simulink model "pattern3x3_training_2023noclock"  (R2024a)
settings: Solver=FixedStepAuto  StartTime=0.0  StopTime=2  FixedStep=0.000005  RelTol=1e-3
model workspace (MAT data in the model file):
  part1_v1 = 1
values from neighbouring files (symbols this model uses):
  full_pattern = load('Pattern4_250.CSV')    [model_setup4.m]
  max_weight2 = 255    [model_setup4.m]
  min_weight2 = 150    [model_setup4.m]
  Th_control_time2 = 0.02    [model_setup4.m]    (also in model_setup_test.m = 2)
  Th_minus_count2 = 10    [model_setup4.m]    (also in model_setup_test.m = 5)
  Th_plus_count2 = 20    [model_setup4.m]    (also in model_setup_test.m)
libraries: simulink x1
(part 4 of 9)

== system pattern3x3_training_2023noclock/Synapse35 ==
  note: weight 초기값
  note: pre spike trace
  note: weight 최댓값
  note: STDP
  note: Synapse
  note: weight 최솟값
  note: post spike trace
  note: 기존 weight + STDP 변화량
  note: weight RC 감소
  Pre_spike : Inport
  addr : Inport  Port=2
  Post_spike : Inport  Port=3
  Add1 : Sum
  Clock1 : Subsystem
  Clock2 : Subsystem
  Clock3 : Subsystem
  Delay1 : Delay  DelayLength=1  SampleTime=0.00001
  Exp : Math
  Exp1 : Math
  From Workspace : FromWorkspace  VariableName=Rand_var
  From Workspace1 : FromWorkspace  VariableName=min_weight
  From Workspace2 : FromWorkspace  VariableName=max_weight
  From Workspace3 : FromWorkspace  VariableName=synapse_weight_rc_s
  From Workspace4 : FromWorkspace  VariableName=synapse_weight_rc_l
  From Workspace6 : FromWorkspace  VariableName=initial_LTP
  From Workspace7 : FromWorkspace  VariableName=initial_LTD
  From Workspace8 : FromWorkspace  VariableName=RC_LTP
  From Workspace9 : FromWorkspace  VariableName=RC_LTD
  Gain1 : Gain  Gain=-1
  MATLAB Function1 : MATLAB Function  TreatAsAtomicUnit=on
  Memory1 : Memory
  Memory2 : Memory
  OR : Logic  Operator=OR  IconShape=distinctive  AllPortsSameDT=off  OutDataTypeStr=boolean
  Product{,1..6} (7 alike) : Product
  Scope1 : Scope  NumInputPorts=4
  Scope2 : Scope  NumInputPorts=5
  Scope3 : Scope  NumInputPorts=2
  Scope5 : Scope  NumInputPorts=3
  Scope6 : Scope  NumInputPorts=3
  Scope7 : Scope  NumInputPorts=3
  Scope8 : Scope  NumInputPorts=4
  Subsystem : Subsystem
  Switch : Switch  Threshold=max_weight2  SaturateOnIntegerOverflow=off  InputSameDT=off
  Switch1 : Switch  Criteria=u2 > Threshold  Threshold=min_weight2  SaturateOnIntegerOverflow=off  InputSameDT=off
  rc_add1 : MATLAB Function  TreatAsAtomicUnit=on
  rc_add2 : MATLAB Function  TreatAsAtomicUnit=on
  Weight : Outport
  Spike_out : Outport  Port=2
  Weight_out : Outport  Port=3
  wires:
  Switch1/1 -> Scope7/3, Product/2, Weight_out/1, Scope5/3, Scope3/1, Delay1/1
  Product/1 -> Memory1/1
  addr/1 -> MATLAB Function1/2(synapse_num)
  Post_spike/1 -> Scope2/4, Memory2/1
  Clock1/1(T) -> rc_add2/1(tx)
  Clock2/1(T) -> Scope2/3, rc_add1/1(ty)
  Delay1/1 -> Scope3/2, Subsystem/2(before_weight), Scope6/3
  Memory1/1 -> Weight/1, Scope5/2
  From Workspace7/1 -> rc_add1/2(initial_LTD)
  From Workspace9/1 -> rc_add1/3(RC_LTD)
  From Workspace6/1 -> rc_add2/2(initial_LTP)
  From Workspace8/1 -> rc_add2/3(RC_LTP)
  Product6/1 -> Scope1/4, Add1/2
  Product5/1 -> Scope1/3, Add1/1
  Add1/1 -> Subsystem/1(delta_weight), Scope2/1, Scope6/1
  From Workspace2/1 -> Product3/2
  Product2/1 -> Exp1/1
  Gain1/1 -> Product1/2, Product2/1
  From Workspace1/1 -> Switch1/3
  Exp1/1 -> Scope8/2, Product4/2
  Switch/1 -> Scope8/4, Switch1/2, Scope7/2, Switch1/1
  From Workspace3/1 -> Product2/2
  Product3/1 -> Switch/1
  Exp/1 -> Product3/1
  Clock3/1(T) -> Gain1/1
  Product1/1 -> Exp/1
  MATLAB Function1/1(y) -> Scope6/2, Product4/1, Scope7/1, Switch/2, Scope8/1
  From Workspace4/1 -> Product1/1
  From Workspace/1 -> MATLAB Function1/1(init_weight)
  Product4/1 -> Scope8/3, Switch/3
  Subsystem/1(weight) -> MATLAB Function1/3(before_weight)
  rc_add2/1(pre_trace) -> Product5/1
  rc_add1/1(post_trace) -> Product6/2
  OR/1 -> Subsystem/Trigger
  Memory2/1 -> OR/2, Scope1/2, Product5/2, Clock2/1("Reset "), Scope2/5
  Pre_spike/1 -> OR/1, Scope1/1, Scope5/1, Spike_out/1, Product/1, Clock3/1("Reset "), Clock1/1("Reset "), Product6/1, Scope2/2

== system pattern3x3_training_2023noclock/Synapse36 ==
  note: weight 초기값
  note: pre spike trace
  note: weight 최댓값
  note: STDP
  note: Synapse
  note: weight 최솟값
  note: post spike trace
  note: 기존 weight + STDP 변화량
  note: weight RC 감소
  Pre_spike : Inport
  addr : Inport  Port=2
  Post_spike : Inport  Port=3
  Add1 : Sum
  Clock1 : Subsystem
  Clock2 : Subsystem
  Clock3 : Subsystem
  Delay1 : Delay  DelayLength=1  SampleTime=0.00001
  Exp : Math
  Exp1 : Math
  From Workspace : FromWorkspace  VariableName=Rand_var
  From Workspace1 : FromWorkspace  VariableName=min_weight
  From Workspace2 : FromWorkspace  VariableName=max_weight
  From Workspace3 : FromWorkspace  VariableName=synapse_weight_rc_s
  From Workspace4 : FromWorkspace  VariableName=synapse_weight_rc_l
  From Workspace6 : FromWorkspace  VariableName=initial_LTP
  From Workspace7 : FromWorkspace  VariableName=initial_LTD
  From Workspace8 : FromWorkspace  VariableName=RC_LTP
  From Workspace9 : FromWorkspace  VariableName=RC_LTD
  Gain1 : Gain  Gain=-1
  MATLAB Function1 : MATLAB Function  TreatAsAtomicUnit=on
  Memory1 : Memory
  Memory2 : Memory
  OR : Logic  Operator=OR  IconShape=distinctive  AllPortsSameDT=off  OutDataTypeStr=boolean
  Product{,1..6} (7 alike) : Product
  Scope1 : Scope  NumInputPorts=4
  Scope2 : Scope  NumInputPorts=5
  Scope3 : Scope  NumInputPorts=2
  Scope5 : Scope  NumInputPorts=3
  Scope6 : Scope  NumInputPorts=3
  Scope7 : Scope  NumInputPorts=3
  Scope8 : Scope  NumInputPorts=4
  Subsystem : Subsystem
  Switch : Switch  Threshold=max_weight2  SaturateOnIntegerOverflow=off  InputSameDT=off
  Switch1 : Switch  Criteria=u2 > Threshold  Threshold=min_weight2  SaturateOnIntegerOverflow=off  InputSameDT=off
  rc_add1 : MATLAB Function  TreatAsAtomicUnit=on
  rc_add2 : MATLAB Function  TreatAsAtomicUnit=on
  Weight : Outport
  Spike_out : Outport  Port=2
  Weight_out : Outport  Port=3
  wires:
  Switch1/1 -> Scope7/3, Product/2, Weight_out/1, Scope5/3, Scope3/1, Delay1/1
  Product/1 -> Memory1/1
  addr/1 -> MATLAB Function1/2(synapse_num)
  Post_spike/1 -> Scope2/4, Memory2/1
  Clock1/1(T) -> rc_add2/1(tx)
  Clock2/1(T) -> Scope2/3, rc_add1/1(ty)
  Delay1/1 -> Scope3/2, Subsystem/2(before_weight), Scope6/3
  Memory1/1 -> Weight/1, Scope5/2
  From Workspace7/1 -> rc_add1/2(initial_LTD)
  From Workspace9/1 -> rc_add1/3(RC_LTD)
  From Workspace6/1 -> rc_add2/2(initial_LTP)
  From Workspace8/1 -> rc_add2/3(RC_LTP)
  Product6/1 -> Scope1/4, Add1/2
  Product5/1 -> Scope1/3, Add1/1
  Add1/1 -> Subsystem/1(delta_weight), Scope2/1, Scope6/1
  From Workspace2/1 -> Product3/2
  Product2/1 -> Exp1/1
  Gain1/1 -> Product1/2, Product2/1
  From Workspace1/1 -> Switch1/3
  Exp1/1 -> Scope8/2, Product4/2
  Switch/1 -> Scope8/4, Switch1/2, Scope7/2, Switch1/1
  From Workspace3/1 -> Product2/2
  Product3/1 -> Switch/1
  Exp/1 -> Product3/1
  Clock3/1(T) -> Gain1/1
  Product1/1 -> Exp/1
  MATLAB Function1/1(y) -> Scope6/2, Product4/1, Scope7/1, Switch/2, Scope8/1
  From Workspace4/1 -> Product1/1
  From Workspace/1 -> MATLAB Function1/1(init_weight)
  Product4/1 -> Scope8/3, Switch/3
  Subsystem/1(weight) -> MATLAB Function1/3(before_weight)
  rc_add2/1(pre_trace) -> Product5/1
  rc_add1/1(post_trace) -> Product6/2
  OR/1 -> Subsystem/Trigger
  Memory2/1 -> OR/2, Scope1/2, Product5/2, Clock2/1("Reset "), Scope2/5
  Pre_spike/1 -> OR/1, Scope1/1, Scope5/1, Spike_out/1, Product/1, Clock3/1("Reset "), Clock1/1("Reset "), Product6/1, Scope2/2

== system pattern3x3_training_2023noclock/Synapse4 ==
  note: weight 초기값
  note: pre spike trace
  note: weight 최댓값
  note: STDP
  note: Synapse
  note: weight 최솟값
  note: post spike trace
  note: 기존 weight + STDP 변화량
  note: weight RC 감소
  Pre_spike : Inport
  addr : Inport  Port=2
  Post_spike : Inport  Port=3
  Add1 : Sum
  Clock1 : Subsystem
  Clock2 : Subsystem
  Clock3 : Subsystem
  Delay1 : Delay  DelayLength=1  SampleTime=0.00001
  Exp : Math
  Exp1 : Math
  From Workspace : FromWorkspace  VariableName=Rand_var
  From Workspace1 : FromWorkspace  VariableName=min_weight
  From Workspace2 : FromWorkspace  VariableName=max_weight
  From Workspace3 : FromWorkspace  VariableName=synapse_weight_rc_s
  From Workspace4 : FromWorkspace  VariableName=synapse_weight_rc_l
  From Workspace6 : FromWorkspace  VariableName=initial_LTP
  From Workspace7 : FromWorkspace  VariableName=initial_LTD
  From Workspace8 : FromWorkspace  VariableName=RC_LTP
  From Workspace9 : FromWorkspace  VariableName=RC_LTD
  Gain1 : Gain  Gain=-1
  MATLAB Function1 : MATLAB Function  TreatAsAtomicUnit=on
  Memory1 : Memory
  Memory2 : Memory
  OR : Logic  Operator=OR  IconShape=distinctive  AllPortsSameDT=off  OutDataTypeStr=boolean
  Product{,1..6} (7 alike) : Product
  Scope1 : Scope  NumInputPorts=4
  Scope2 : Scope  NumInputPorts=5
  Scope3 : Scope  NumInputPorts=2
  Scope5 : Scope  NumInputPorts=3
  Scope6 : Scope  NumInputPorts=3
  Scope7 : Scope  NumInputPorts=3
  Scope8 : Scope  NumInputPorts=4
  Subsystem : Subsystem
  Switch : Switch  Threshold=max_weight2  SaturateOnIntegerOverflow=off  InputSameDT=off
  Switch1 : Switch  Criteria=u2 > Threshold  Threshold=min_weight2  SaturateOnIntegerOverflow=off  InputSameDT=off
  rc_add1 : MATLAB Function  TreatAsAtomicUnit=on
  rc_add2 : MATLAB Function  TreatAsAtomicUnit=on
  Weight : Outport
  Spike_out : Outport  Port=2
  Weight_out : Outport  Port=3
  wires:
  Switch1/1 -> Scope7/3, Product/2, Weight_out/1, Scope5/3, Scope3/1, Delay1/1
  Product/1 -> Memory1/1
  addr/1 -> MATLAB Function1/2(synapse_num)
  Post_spike/1 -> Scope2/4, Memory2/1
  Clock1/1(T) -> rc_add2/1(tx)
  Clock2/1(T) -> Scope2/3, rc_add1/1(ty)
  Delay1/1 -> Scope3/2, Subsystem/2(before_weight), Scope6/3
  Memory1/1 -> Weight/1, Scope5/2
  From Workspace7/1 -> rc_add1/2(initial_LTD)
  From Workspace9/1 -> rc_add1/3(RC_LTD)
  From Workspace6/1 -> rc_add2/2(initial_LTP)
  From Workspace8/1 -> rc_add2/3(RC_LTP)
  Product6/1 -> Scope1/4, Add1/2
  Product5/1 -> Scope1/3, Add1/1
  Add1/1 -> Subsystem/1(delta_weight), Scope2/1, Scope6/1
  From Workspace2/1 -> Product3/2
  Product2/1 -> Exp1/1
  Gain1/1 -> Product1/2, Product2/1
  From Workspace1/1 -> Switch1/3
  Exp1/1 -> Scope8/2, Product4/2
  Switch/1 -> Scope8/4, Switch1/2, Scope7/2, Switch1/1
  From Workspace3/1 -> Product2/2
  Product3/1 -> Switch/1
  Exp/1 -> Product3/1
  Clock3/1(T) -> Gain1/1
  Product1/1 -> Exp/1
  MATLAB Function1/1(y) -> Scope6/2, Product4/1, Scope7/1, Switch/2, Scope8/1
  From Workspace4/1 -> Product1/1
  From Workspace/1 -> MATLAB Function1/1(init_weight)
  Product4/1 -> Scope8/3, Switch/3
  Subsystem/1(weight) -> MATLAB Function1/3(before_weight)
  rc_add2/1(pre_trace) -> Product5/1
  rc_add1/1(post_trace) -> Product6/2
  OR/1 -> Subsystem/Trigger
  Memory2/1 -> OR/2, Scope1/2, Product5/2, Clock2/1("Reset "), Scope2/5
  Pre_spike/1 -> OR/1, Scope1/1, Scope5/1, Spike_out/1, Product/1, Clock3/1("Reset "), Clock1/1("Reset "), Product6/1, Scope2/2

== system pattern3x3_training_2023noclock/Synapse5 ==
  note: weight 초기값
  note: pre spike trace
  note: weight 최댓값
  note: STDP
  note: Synapse
  note: weight 최솟값
  note: post spike trace
  note: 기존 weight + STDP 변화량
  note: weight RC 감소
  Pre_spike : Inport
  addr : Inport  Port=2
  Post_spike : Inport  Port=3
  Add1 : Sum
  Clock1 : Subsystem
  Clock2 : Subsystem
  Clock3 : Subsystem
  Delay1 : Delay  DelayLength=1  SampleTime=0.00001
  Exp : Math
  Exp1 : Math
  From Workspace : FromWorkspace  VariableName=Rand_var
  From Workspace1 : FromWorkspace  VariableName=min_weight
  From Workspace2 : FromWorkspace  VariableName=max_weight
  From Workspace3 : FromWorkspace  VariableName=synapse_weight_rc_s
  From Workspace4 : FromWorkspace  VariableName=synapse_weight_rc_l
  From Workspace6 : FromWorkspace  VariableName=initial_LTP
  From Workspace7 : FromWorkspace  VariableName=initial_LTD
  From Workspace8 : FromWorkspace  VariableName=RC_LTP
  From Workspace9 : FromWorkspace  VariableName=RC_LTD
  Gain1 : Gain  Gain=-1
  MATLAB Function1 : MATLAB Function  TreatAsAtomicUnit=on
  Memory1 : Memory
  Memory2 : Memory
  OR : Logic  Operator=OR  IconShape=distinctive  AllPortsSameDT=off  OutDataTypeStr=boolean
  Product{,1..6} (7 alike) : Product
  Scope1 : Scope  NumInputPorts=4
  Scope2 : Scope  NumInputPorts=5
  Scope3 : Scope  NumInputPorts=2
  Scope5 : Scope  NumInputPorts=3
  Scope6 : Scope  NumInputPorts=3
  Scope7 : Scope  NumInputPorts=3
  Scope8 : Scope  NumInputPorts=4
  Subsystem : Subsystem
  Switch : Switch  Threshold=max_weight2  SaturateOnIntegerOverflow=off  InputSameDT=off
  Switch1 : Switch  Criteria=u2 > Threshold  Threshold=min_weight2  SaturateOnIntegerOverflow=off  InputSameDT=off
  rc_add1 : MATLAB Function  TreatAsAtomicUnit=on
  rc_add2 : MATLAB Function  TreatAsAtomicUnit=on
  Weight : Outport
  Spike_out : Outport  Port=2
  Weight_out : Outport  Port=3
  wires:
  Switch1/1 -> Scope7/3, Product/2, Weight_out/1, Scope5/3, Scope3/1, Delay1/1
  Product/1 -> Memory1/1
  addr/1 -> MATLAB Function1/2(synapse_num)
  Post_spike/1 -> Scope2/4, Memory2/1
  Clock1/1(T) -> rc_add2/1(tx)
  Clock2/1(T) -> Scope2/3, rc_add1/1(ty)
  Delay1/1 -> Scope3/2, Subsystem/2(before_weight), Scope6/3
  Memory1/1 -> Weight/1, Scope5/2
  From Workspace7/1 -> rc_add1/2(initial_LTD)
  From Workspace9/1 -> rc_add1/3(RC_LTD)
  From Workspace6/1 -> rc_add2/2(initial_LTP)
  From Workspace8/1 -> rc_add2/3(RC_LTP)
  Product6/1 -> Scope1/4, Add1/2
  Product5/1 -> Scope1/3, Add1/1
  Add1/1 -> Subsystem/1(delta_weight), Scope2/1, Scope6/1
  From Workspace2/1 -> Product3/2
  Product2/1 -> Exp1/1
  Gain1/1 -> Product1/2, Product2/1
  From Workspace1/1 -> Switch1/3
  Exp1/1 -> Scope8/2, Product4/2
  Switch/1 -> Scope8/4, Switch1/2, Scope7/2, Switch1/1
  From Workspace3/1 -> Product2/2
  Product3/1 -> Switch/1
  Exp/1 -> Product3/1
  Clock3/1(T) -> Gain1/1
  Product1/1 -> Exp/1
  MATLAB Function1/1(y) -> Scope6/2, Product4/1, Scope7/1, Switch/2, Scope8/1
  From Workspace4/1 -> Product1/1
  From Workspace/1 -> MATLAB Function1/1(init_weight)
  Product4/1 -> Scope8/3, Switch/3
  Subsystem/1(weight) -> MATLAB Function1/3(before_weight)
  rc_add2/1(pre_trace) -> Product5/1
  rc_add1/1(post_trace) -> Product6/2
  OR/1 -> Subsystem/Trigger
  Memory2/1 -> OR/2, Scope1/2, Product5/2, Clock2/1("Reset "), Scope2/5
  Pre_spike/1 -> OR/1, Scope1/1, Scope5/1, Spike_out/1, Product/1, Clock3/1("Reset "), Clock1/1("Reset "), Product6/1, Scope2/2

== system pattern3x3_training_2023noclock/Synapse6 ==
  note: weight 초기값
  note: pre spike trace
  note: weight 최댓값
  note: STDP
  note: Synapse
  note: weight 최솟값
  note: post spike trace
  note: 기존 weight + STDP 변화량
  note: weight RC 감소
  Pre_spike : Inport
  addr : Inport  Port=2
  Post_spike : Inport  Port=3
  Add1 : Sum
  Clock1 : Subsystem
  Clock2 : Subsystem
  Clock3 : Subsystem
  Delay1 : Delay  DelayLength=1  SampleTime=0.00001
  Exp : Math
  Exp1 : Math
  From Workspace : FromWorkspace  VariableName=Rand_var
  From Workspace1 : FromWorkspace  VariableName=min_weight
  From Workspace2 : FromWorkspace  VariableName=max_weight
  From Workspace3 : FromWorkspace  VariableName=synapse_weight_rc_s
  From Workspace4 : FromWorkspace  VariableName=synapse_weight_rc_l
  From Workspace6 : FromWorkspace  VariableName=initial_LTP
  From Workspace7 : FromWorkspace  VariableName=initial_LTD
  From Workspace8 : FromWorkspace  VariableName=RC_LTP
  From Workspace9 : FromWorkspace  VariableName=RC_LTD
  Gain1 : Gain  Gain=-1
  MATLAB Function1 : MATLAB Function  TreatAsAtomicUnit=on
  Memory1 : Memory
  Memory2 : Memory
  OR : Logic  Operator=OR  IconShape=distinctive  AllPortsSameDT=off  OutDataTypeStr=boolean
  Product{,1..6} (7 alike) : Product
  Scope1 : Scope  NumInputPorts=4
  Scope2 : Scope  NumInputPorts=5
  Scope3 : Scope  NumInputPorts=2
  Scope5 : Scope  NumInputPorts=3
  Scope6 : Scope  NumInputPorts=3
  Scope7 : Scope  NumInputPorts=3
  Scope8 : Scope  NumInputPorts=4
  Subsystem : Subsystem
  Switch : Switch  Threshold=max_weight2  SaturateOnIntegerOverflow=off  InputSameDT=off
  Switch1 : Switch  Criteria=u2 > Threshold  Threshold=min_weight2  SaturateOnIntegerOverflow=off  InputSameDT=off
  rc_add1 : MATLAB Function  TreatAsAtomicUnit=on
  rc_add2 : MATLAB Function  TreatAsAtomicUnit=on
  Weight : Outport
  Spike_out : Outport  Port=2
  Weight_out : Outport  Port=3
  wires:
  Switch1/1 -> Scope7/3, Product/2, Weight_out/1, Scope5/3, Scope3/1, Delay1/1
  Product/1 -> Memory1/1
  addr/1 -> MATLAB Function1/2(synapse_num)
  Post_spike/1 -> Scope2/4, Memory2/1
  Clock1/1(T) -> rc_add2/1(tx)
  Clock2/1(T) -> Scope2/3, rc_add1/1(ty)
  Delay1/1 -> Scope3/2, Subsystem/2(before_weight), Scope6/3
  Memory1/1 -> Weight/1, Scope5/2
  From Workspace7/1 -> rc_add1/2(initial_LTD)
  From Workspace9/1 -> rc_add1/3(RC_LTD)
  From Workspace6/1 -> rc_add2/2(initial_LTP)
  From Workspace8/1 -> rc_add2/3(RC_LTP)
  Product6/1 -> Scope1/4, Add1/2
  Product5/1 -> Scope1/3, Add1/1
  Add1/1 -> Subsystem/1(delta_weight), Scope2/1, Scope6/1
  From Workspace2/1 -> Product3/2
  Product2/1 -> Exp1/1
  Gain1/1 -> Product1/2, Product2/1
  From Workspace1/1 -> Switch1/3
  Exp1/1 -> Scope8/2, Product4/2
  Switch/1 -> Scope8/4, Switch1/2, Scope7/2, Switch1/1
  From Workspace3/1 -> Product2/2
  Product3/1 -> Switch/1
  Exp/1 -> Product3/1
  Clock3/1(T) -> Gain1/1
  Product1/1 -> Exp/1
  MATLAB Function1/1(y) -> Scope6/2, Product4/1, Scope7/1, Switch/2, Scope8/1
  From Workspace4/1 -> Product1/1
  From Workspace/1 -> MATLAB Function1/1(init_weight)
  Product4/1 -> Scope8/3, Switch/3
  Subsystem/1(weight) -> MATLAB Function1/3(before_weight)
  rc_add2/1(pre_trace) -> Product5/1
  rc_add1/1(post_trace) -> Product6/2
  OR/1 -> Subsystem/Trigger
  Memory2/1 -> OR/2, Scope1/2, Product5/2, Clock2/1("Reset "), Scope2/5
  Pre_spike/1 -> OR/1, Scope1/1, Scope5/1, Spike_out/1, Product/1, Clock3/1("Reset "), Clock1/1("Reset "), Product6/1, Scope2/2

== system pattern3x3_training_2023noclock/Synapse7 ==
  note: weight 초기값
  note: pre spike trace
  note: weight 최댓값
  note: STDP
  note: Synapse
  note: weight 최솟값
  note: post spike trace
  note: 기존 weight + STDP 변화량
  note: weight RC 감소
  Pre_spike : Inport
  addr : Inport  Port=2
  Post_spike : Inport  Port=3
  Add1 : Sum
  Clock1 : Subsystem
  Clock2 : Subsystem
  Clock3 : Subsystem
  Delay1 : Delay  DelayLength=1  SampleTime=0.00001
  Exp : Math
  Exp1 : Math
  From Workspace : FromWorkspace  VariableName=Rand_var
  From Workspace1 : FromWorkspace  VariableName=min_weight
  From Workspace2 : FromWorkspace  VariableName=max_weight
  From Workspace3 : FromWorkspace  VariableName=synapse_weight_rc_s
  From Workspace4 : FromWorkspace  VariableName=synapse_weight_rc_l
  From Workspace6 : FromWorkspace  VariableName=initial_LTP
  From Workspace7 : FromWorkspace  VariableName=initial_LTD
  From Workspace8 : FromWorkspace  VariableName=RC_LTP
  From Workspace9 : FromWorkspace  VariableName=RC_LTD
  Gain1 : Gain  Gain=-1
  MATLAB Function1 : MATLAB Function  TreatAsAtomicUnit=on
  Memory1 : Memory
  Memory2 : Memory
  OR : Logic  Operator=OR  IconShape=distinctive  AllPortsSameDT=off  OutDataTypeStr=boolean
  Product{,1..6} (7 alike) : Product
  Scope1 : Scope  NumInputPorts=4
  Scope2 : Scope  NumInputPorts=5
  Scope3 : Scope  NumInputPorts=2
  Scope5 : Scope  NumInputPorts=3
  Scope6 : Scope  NumInputPorts=3
  Scope7 : Scope  NumInputPorts=3
  Scope8 : Scope  NumInputPorts=4
  Subsystem : Subsystem
  Switch : Switch  Threshold=max_weight2  SaturateOnIntegerOverflow=off  InputSameDT=off
  Switch1 : Switch  Criteria=u2 > Threshold  Threshold=min_weight2  SaturateOnIntegerOverflow=off  InputSameDT=off
  rc_add1 : MATLAB Function  TreatAsAtomicUnit=on
  rc_add2 : MATLAB Function  TreatAsAtomicUnit=on
  Weight : Outport
  Spike_out : Outport  Port=2
  Weight_out : Outport  Port=3
  wires:
  Switch1/1 -> Scope7/3, Product/2, Weight_out/1, Scope5/3, Scope3/1, Delay1/1
  Product/1 -> Memory1/1
  addr/1 -> MATLAB Function1/2(synapse_num)
  Post_spike/1 -> Scope2/4, Memory2/1
  Clock1/1(T) -> rc_add2/1(tx)
  Clock2/1(T) -> Scope2/3, rc_add1/1(ty)
  Delay1/1 -> Scope3/2, Subsystem/2(before_weight), Scope6/3
  Memory1/1 -> Weight/1, Scope5/2
  From Workspace7/1 -> rc_add1/2(initial_LTD)
  From Workspace9/1 -> rc_add1/3(RC_LTD)
  From Workspace6/1 -> rc_add2/2(initial_LTP)
  From Workspace8/1 -> rc_add2/3(RC_LTP)
  Product6/1 -> Scope1/4, Add1/2
  Product5/1 -> Scope1/3, Add1/1
  Add1/1 -> Subsystem/1(delta_weight), Scope2/1, Scope6/1
  From Workspace2/1 -> Product3/2
  Product2/1 -> Exp1/1
  Gain1/1 -> Product1/2, Product2/1
  From Workspace1/1 -> Switch1/3
  Exp1/1 -> Scope8/2, Product4/2
  Switch/1 -> Scope8/4, Switch1/2, Scope7/2, Switch1/1
  From Workspace3/1 -> Product2/2
  Product3/1 -> Switch/1
  Exp/1 -> Product3/1
  Clock3/1(T) -> Gain1/1
  Product1/1 -> Exp/1
  MATLAB Function1/1(y) -> Scope6/2, Product4/1, Scope7/1, Switch/2, Scope8/1
  From Workspace4/1 -> Product1/1
  From Workspace/1 -> MATLAB Function1/1(init_weight)
  Product4/1 -> Scope8/3, Switch/3
  Subsystem/1(weight) -> MATLAB Function1/3(before_weight)
  rc_add2/1(pre_trace) -> Product5/1
  rc_add1/1(post_trace) -> Product6/2
  OR/1 -> Subsystem/Trigger
  Memory2/1 -> OR/2, Scope1/2, Product5/2, Clock2/1("Reset "), Scope2/5
  Pre_spike/1 -> OR/1, Scope1/1, Scope5/1, Spike_out/1, Product/1, Clock3/1("Reset "), Clock1/1("Reset "), Product6/1, Scope2/2

== system pattern3x3_training_2023noclock/Synapse8 ==
  note: weight 초기값
  note: pre spike trace
  note: weight 최댓값
  note: STDP
  note: Synapse
  note: weight 최솟값
  note: post spike trace
  note: 기존 weight + STDP 변화량
  note: weight RC 감소
  Pre_spike : Inport
  addr : Inport  Port=2
  Post_spike : Inport  Port=3
  Add1 : Sum
  Clock1 : Subsystem
  Clock2 : Subsystem
  Clock3 : Subsystem
  Delay1 : Delay  DelayLength=1  SampleTime=0.00001
  Exp : Math
  Exp1 : Math
  From Workspace : FromWorkspace  VariableName=Rand_var
  From Workspace1 : FromWorkspace  VariableName=min_weight
  From Workspace2 : FromWorkspace  VariableName=max_weight
  From Workspace3 : FromWorkspace  VariableName=synapse_weight_rc_s
  From Workspace4 : FromWorkspace  VariableName=synapse_weight_rc_l
  From Workspace6 : FromWorkspace  VariableName=initial_LTP
  From Workspace7 : FromWorkspace  VariableName=initial_LTD
  From Workspace8 : FromWorkspace  VariableName=RC_LTP
  From Workspace9 : FromWorkspace  VariableName=RC_LTD
  Gain1 : Gain  Gain=-1
  MATLAB Function1 : MATLAB Function  TreatAsAtomicUnit=on
  Memory1 : Memory
  Memory2 : Memory
  OR : Logic  Operator=OR  IconShape=distinctive  AllPortsSameDT=off  OutDataTypeStr=boolean
  Product{,1..6} (7 alike) : Product
  Scope1 : Scope  NumInputPorts=4
  Scope2 : Scope  NumInputPorts=5
  Scope3 : Scope  NumInputPorts=2
  Scope5 : Scope  NumInputPorts=3
  Scope6 : Scope  NumInputPorts=3
  Scope7 : Scope  NumInputPorts=3
  Scope8 : Scope  NumInputPorts=4
  Subsystem : Subsystem
  Switch : Switch  Threshold=max_weight2  SaturateOnIntegerOverflow=off  InputSameDT=off
  Switch1 : Switch  Criteria=u2 > Threshold  Threshold=min_weight2  SaturateOnIntegerOverflow=off  InputSameDT=off
  rc_add1 : MATLAB Function  TreatAsAtomicUnit=on
  rc_add2 : MATLAB Function  TreatAsAtomicUnit=on
  Weight : Outport
  Spike_out : Outport  Port=2
  Weight_out : Outport  Port=3
  wires:
  Switch1/1 -> Scope7/3, Product/2, Weight_out/1, Scope5/3, Scope3/1, Delay1/1
  Product/1 -> Memory1/1
  addr/1 -> MATLAB Function1/2(synapse_num)
  Post_spike/1 -> Scope2/4, Memory2/1
  Clock1/1(T) -> rc_add2/1(tx)
  Clock2/1(T) -> Scope2/3, rc_add1/1(ty)
  Delay1/1 -> Scope3/2, Subsystem/2(before_weight), Scope6/3
  Memory1/1 -> Weight/1, Scope5/2
  From Workspace7/1 -> rc_add1/2(initial_LTD)
  From Workspace9/1 -> rc_add1/3(RC_LTD)
  From Workspace6/1 -> rc_add2/2(initial_LTP)
  From Workspace8/1 -> rc_add2/3(RC_LTP)
  Product6/1 -> Scope1/4, Add1/2
  Product5/1 -> Scope1/3, Add1/1
  Add1/1 -> Subsystem/1(delta_weight), Scope2/1, Scope6/1
  From Workspace2/1 -> Product3/2
  Product2/1 -> Exp1/1
  Gain1/1 -> Product1/2, Product2/1
  From Workspace1/1 -> Switch1/3
  Exp1/1 -> Scope8/2, Product4/2
  Switch/1 -> Scope8/4, Switch1/2, Scope7/2, Switch1/1
  From Workspace3/1 -> Product2/2
  Product3/1 -> Switch/1
  Exp/1 -> Product3/1
  Clock3/1(T) -> Gain1/1
  Product1/1 -> Exp/1
  MATLAB Function1/1(y) -> Scope6/2, Product4/1, Scope7/1, Switch/2, Scope8/1
  From Workspace4/1 -> Product1/1
  From Workspace/1 -> MATLAB Function1/1(init_weight)
  Product4/1 -> Scope8/3, Switch/3
  Subsystem/1(weight) -> MATLAB Function1/3(before_weight)
  rc_add2/1(pre_trace) -> Product5/1
  rc_add1/1(post_trace) -> Product6/2
  OR/1 -> Subsystem/Trigger
  Memory2/1 -> OR/2, Scope1/2, Product5/2, Clock2/1("Reset "), Scope2/5
  Pre_spike/1 -> OR/1, Scope1/1, Scope5/1, Spike_out/1, Product/1, Clock3/1("Reset "), Clock1/1("Reset "), Product6/1, Scope2/2

== system pattern3x3_training_2023noclock/Synapse9 ==
  note: weight 초기값
  note: pre spike trace
  note: weight 최댓값
  note: STDP
  note: Synapse
  note: weight 최솟값
  note: post spike trace
  note: 기존 weight + STDP 변화량
  note: weight RC 감소
  Pre_spike : Inport
  addr : Inport  Port=2
  Post_spike : Inport  Port=3
  Add1 : Sum
  Clock1 : Subsystem
  Clock2 : Subsystem
  Clock3 : Subsystem
  Delay1 : Delay  DelayLength=1  SampleTime=0.00001
  Exp : Math
  Exp1 : Math
  From Workspace : FromWorkspace  VariableName=Rand_var
  From Workspace1 : FromWorkspace  VariableName=min_weight
  From Workspace2 : FromWorkspace  VariableName=max_weight
  From Workspace3 : FromWorkspace  VariableName=synapse_weight_rc_s
  From Workspace4 : FromWorkspace  VariableName=synapse_weight_rc_l
  From Workspace6 : FromWorkspace  VariableName=initial_LTP
  From Workspace7 : FromWorkspace  VariableName=initial_LTD
  From Workspace8 : FromWorkspace  VariableName=RC_LTP
  From Workspace9 : FromWorkspace  VariableName=RC_LTD
  Gain1 : Gain  Gain=-1
  MATLAB Function1 : MATLAB Function  TreatAsAtomicUnit=on
  Memory1 : Memory
  Memory2 : Memory
  OR : Logic  Operator=OR  IconShape=distinctive  AllPortsSameDT=off  OutDataTypeStr=boolean
  Product{,1..6} (7 alike) : Product
  Scope1 : Scope  NumInputPorts=4
  Scope2 : Scope  NumInputPorts=5
  Scope3 : Scope  NumInputPorts=2
  Scope5 : Scope  NumInputPorts=3
  Scope6 : Scope  NumInputPorts=3
  Scope7 : Scope  NumInputPorts=3
  Scope8 : Scope  NumInputPorts=4
  Subsystem : Subsystem
  Switch : Switch  Threshold=max_weight2  SaturateOnIntegerOverflow=off  InputSameDT=off
  Switch1 : Switch  Criteria=u2 > Threshold  Threshold=min_weight2  SaturateOnIntegerOverflow=off  InputSameDT=off
  rc_add1 : MATLAB Function  TreatAsAtomicUnit=on
  rc_add2 : MATLAB Function  TreatAsAtomicUnit=on
  Weight : Outport
  Spike_out : Outport  Port=2
  Weight_out : Outport  Port=3
  wires:
  Switch1/1 -> Scope7/3, Product/2, Weight_out/1, Scope5/3, Scope3/1, Delay1/1
  Product/1 -> Memory1/1
  addr/1 -> MATLAB Function1/2(synapse_num)
  Post_spike/1 -> Scope2/4, Memory2/1
  Clock1/1(T) -> rc_add2/1(tx)
  Clock2/1(T) -> Scope2/3, rc_add1/1(ty)
  Delay1/1 -> Scope3/2, Subsystem/2(before_weight), Scope6/3
  Memory1/1 -> Weight/1, Scope5/2
  From Workspace7/1 -> rc_add1/2(initial_LTD)
  From Workspace9/1 -> rc_add1/3(RC_LTD)
  From Workspace6/1 -> rc_add2/2(initial_LTP)
  From Workspace8/1 -> rc_add2/3(RC_LTP)
  Product6/1 -> Scope1/4, Add1/2
  Product5/1 -> Scope1/3, Add1/1
  Add1/1 -> Subsystem/1(delta_weight), Scope2/1, Scope6/1
  From Workspace2/1 -> Product3/2
  Product2/1 -> Exp1/1
  Gain1/1 -> Product1/2, Product2/1
  From Workspace1/1 -> Switch1/3
  Exp1/1 -> Scope8/2, Product4/2
  Switch/1 -> Scope8/4, Switch1/2, Scope7/2, Switch1/1
  From Workspace3/1 -> Product2/2
  Product3/1 -> Switch/1
  Exp/1 -> Product3/1
  Clock3/1(T) -> Gain1/1
  Product1/1 -> Exp/1
  MATLAB Function1/1(y) -> Scope6/2, Product4/1, Scope7/1, Switch/2, Scope8/1
  From Workspace4/1 -> Product1/1
  From Workspace/1 -> MATLAB Function1/1(init_weight)
  Product4/1 -> Scope8/3, Switch/3
  Subsystem/1(weight) -> MATLAB Function1/3(before_weight)
  rc_add2/1(pre_trace) -> Product5/1
  rc_add1/1(post_trace) -> Product6/2
  OR/1 -> Subsystem/Trigger
  Memory2/1 -> OR/2, Scope1/2, Product5/2, Clock2/1("Reset "), Scope2/5
  Pre_spike/1 -> OR/1, Scope1/1, Scope5/1, Spike_out/1, Product/1, Clock3/1("Reset "), Clock1/1("Reset "), Product6/1, Scope2/2

== system pattern3x3_training_2023noclock/Neuron1/Clock4 ==
  "Reset " : Inport
  Memory2 : Memory
  NOT1 : Logic  Operator=NOT  IconShape=distinctive  AllPortsSameDT=off  OutDataTypeStr=boolean
  Product1 : Product
  Pulse Generator1 : DiscretePulseGenerator  PulseType=Time based  Period=0.00001  PulseWidth=50
  Triggered Subsystem1 : Subsystem  TreatAsAtomicUnit=on
  T : Outport  VectorParamsAs1DForOutWhenUnconnected=off
  wires:
  Memory2/1 -> Triggered Subsystem1/1(In1)
  Product1/1 -> T/1, Memory2/1
  Pulse Generator1/1 -> Triggered Subsystem1/Trigger
  "Reset "/1 -> NOT1/1
  Triggered Subsystem1/1(Out1) -> Product1/1
  NOT1/1 -> Product1/2

== system pattern3x3_training_2023noclock/Neuron1/Clock5 ==
  "Reset " : Inport
  Memory2 : Memory
  NOT1 : Logic  Operator=NOT  IconShape=distinctive  AllPortsSameDT=off  OutDataTypeStr=boolean
  Product1 : Product
  Pulse Generator1 : DiscretePulseGenerator  PulseType=Time based  Period=0.00001  PulseWidth=50
  Triggered Subsystem1 : Subsystem  TreatAsAtomicUnit=on
  T : Outport  VectorParamsAs1DForOutWhenUnconnected=off
  wires:
  Memory2/1 -> Triggered Subsystem1/1(In1)
  Product1/1 -> T/1, Memory2/1
  Pulse Generator1/1 -> Triggered Subsystem1/Trigger
  "Reset "/1 -> NOT1/1
  Triggered Subsystem1/1(Out1) -> Product1/1
  NOT1/1 -> Product1/2

== system pattern3x3_training_2023noclock/Neuron1/Subsystem2 ==
  note: 기존 membrane potential + input potential
  Input potential : Inport
  before_Potential : Inport  Port=2
  Trigger : TriggerPort  VariantControl=(inherit)  PortDimensions=1
  Sum : Sum  Inputs=|++
  membrane_state : Outport
  wires:
  Input potential/1 -> Sum/1
  Sum/1 -> membrane_state/1
  before_Potential/1 -> Sum/2

== system pattern3x3_training_2023noclock/Neuron1/Subsystem3 ==
  spike : Inport  OutDataTypeStr=double
  initial_threshold : Inport  Port=2
  neuron_num : Inport  Port=3
  Add1 : Sum
  Constant2 : Constant  Value=0
  Delay : Delay  DelayLength=1  SampleTime=0.00001
  Delay1 : Delay  DelayLength=1  SampleTime=0.00001
  From Workspace3 : FromWorkspace  VariableName=Th_plus
  From Workspace4 : FromWorkspace  VariableName=Th_minus
  From Workspace5 : FromWorkspace  VariableName=Th_mean_count
  From Workspace6 : FromWorkspace  VariableName=min_th
  From Workspace7 : FromWorkspace  VariableName=max_th
  MATLAB Function : MATLAB Function  TreatAsAtomicUnit=on
  MATLAB Function2 : MATLAB Function  TreatAsAtomicUnit=on
  Memory2 : Memory
  NOT : Logic  Operator=NOT  IconShape=distinctive  AllPortsSameDT=off  OutDataTypeStr=boolean
  Product : Product
  Product1 : Product
  Pulse Generator5 : DiscretePulseGenerator  PulseType=Time based  Period=Th_control_time2  PulseWidth=0.00001/Th_control_time2*100  PhaseDelay=Th_control_time2
  Scope1 : Scope  NumInputPorts=3
  Scope2 : Scope  NumInputPorts=3
  Scope3 : Scope  NumInputPorts=3
  Scope4 : Scope  NumInputPorts=4
  Sum : Sum  Inputs=++|
  Sum1 : Sum  Inputs=|++
  Switch3 : Switch  Criteria=u2 > Threshold  SaturateOnIntegerOverflow=off  InputSameDT=off
  Switch4 : Switch  Threshold=Th_plus_count2  SaturateOnIntegerOverflow=off  InputSameDT=off
  Switch5 : Switch  Threshold=Th_minus_count2  SaturateOnIntegerOverflow=off  InputSameDT=off
  spike_generator2 : Subsystem
  Threshold : Outport
  wires:
  MATLAB Function2/1(y) -> Scope3/1, Sum/2
  Sum/1 -> MATLAB Function/1(u)  "Threshold"
  From Workspace7/1 -> MATLAB Function/3(max)
  Delay1/1 -> Scope3/3, MATLAB Function2/3(before_threshold)
  neuron_num/1 -> MATLAB Function2/2(neuron_num)
  MATLAB Function/1(y) -> Delay1/1, Scope3/2, Threshold/1
  initial_threshold/1 -> MATLAB Function2/1(init_th)
  From Workspace6/1 -> MATLAB Function/2(min)
  Pulse Generator5/1 -> Switch3/2, Scope4/1, Product1/1, NOT/1
  Product1/1 -> Scope2/2, Scope4/2, spike_generator2/1(del_th)
  spike/1 -> Scope2/1, Sum1/1
  Delay/1 -> Sum1/2
  Product/1 -> Delay/1, Scope2/3
  Switch4/1 -> Add1/1, Scope1/1
  Switch5/1 -> Scope1/3, Add1/2
  Sum1/1 -> Product1/2, Product/2
  Constant2/1 -> Switch5/1, Switch4/3
  From Workspace4/1 -> Switch5/3
  Switch3/1 -> Scope4/4, Switch5/2, Switch4/2
  From Workspace3/1 -> Switch4/1
  NOT/1 -> Product/1
  spike_generator2/1(del_th_spike) -> Switch3/1, Scope4/3
  From Workspace5/1 -> Switch3/3
  Memory2/1 -> Scope1/2, Sum/1
  Add1/1 -> Memory2/1

== system pattern3x3_training_2023noclock/Neuron1/spike_generator1 ==
  1 : Inport
  AND : Logic  IconShape=distinctive  AllPortsSameDT=off  OutDataTypeStr=boolean
  Cast To Double : DataTypeConversion  OutDataTypeStr=double  SaturateOnIntegerOverflow=off  RndMeth=Floor
  Delay1 : Delay
  NOT : Logic  Operator=NOT  IconShape=distinctive  AllPortsSameDT=off  OutDataTypeStr=boolean
  Scope3 : Scope  NumInputPorts=5
  spike : Outport
  wires:
  NOT/1 -> Scope3/2, Delay1/1
  Delay1/1 -> Scope3/3, AND/2
  AND/1 -> Scope3/4, Cast To Double/1
  1/1 -> AND/1, Scope3/1, NOT/1
  Cast To Double/1 -> Scope3/5, spike/1

== system pattern3x3_training_2023noclock/Neuron2/Clock4 ==
  "Reset " : Inport
  Memory2 : Memory
  NOT1 : Logic  Operator=NOT  IconShape=distinctive  AllPortsSameDT=off  OutDataTypeStr=boolean
  Product1 : Product
  Pulse Generator1 : DiscretePulseGenerator  PulseType=Time based  Period=0.00001  PulseWidth=50
  Triggered Subsystem1 : Subsystem  TreatAsAtomicUnit=on
  T : Outport  VectorParamsAs1DForOutWhenUnconnected=off
  wires:
  Memory2/1 -> Triggered Subsystem1/1(In1)
  Product1/1 -> T/1, Memory2/1
  Pulse Generator1/1 -> Triggered Subsystem1/Trigger
  "Reset "/1 -> NOT1/1
  Triggered Subsystem1/1(Out1) -> Product1/1
  NOT1/1 -> Product1/2

== system pattern3x3_training_2023noclock/Neuron2/Clock5 ==
  "Reset " : Inport
  Memory2 : Memory
  NOT1 : Logic  Operator=NOT  IconShape=distinctive  AllPortsSameDT=off  OutDataTypeStr=boolean
  Product1 : Product
  Pulse Generator1 : DiscretePulseGenerator  PulseType=Time based  Period=0.00001  PulseWidth=50
  Triggered Subsystem1 : Subsystem  TreatAsAtomicUnit=on
  T : Outport  VectorParamsAs1DForOutWhenUnconnected=off
  wires:
  Memory2/1 -> Triggered Subsystem1/1(In1)
  Product1/1 -> T/1, Memory2/1
  Pulse Generator1/1 -> Triggered Subsystem1/Trigger
  "Reset "/1 -> NOT1/1
  Triggered Subsystem1/1(Out1) -> Product1/1
  NOT1/1 -> Product1/2

== system pattern3x3_training_2023noclock/Neuron2/Subsystem2 ==
  note: 기존 membrane potential + input potential
  Input potential : Inport
  before_Potential : Inport  Port=2
  Trigger : TriggerPort  VariantControl=(inherit)  PortDimensions=1
  Sum : Sum  Inputs=|++
  membrane_state : Outport
  wires:
  Input potential/1 -> Sum/1
  Sum/1 -> membrane_state/1
  before_Potential/1 -> Sum/2

== system pattern3x3_training_2023noclock/Neuron2/Subsystem3 ==
  spike : Inport  OutDataTypeStr=double
  initial_threshold : Inport  Port=2
  neuron_num : Inport  Port=3
  Add1 : Sum
  Constant2 : Constant  Value=0
  Delay : Delay  DelayLength=1  SampleTime=0.00001
  Delay1 : Delay  DelayLength=1  SampleTime=0.00001
  From Workspace3 : FromWorkspace  VariableName=Th_plus
  From Workspace4 : FromWorkspace  VariableName=Th_minus
  From Workspace5 : FromWorkspace  VariableName=Th_mean_count
  From Workspace6 : FromWorkspace  VariableName=min_th
  From Workspace7 : FromWorkspace  VariableName=max_th
  MATLAB Function : MATLAB Function  TreatAsAtomicUnit=on
  MATLAB Function2 : MATLAB Function  TreatAsAtomicUnit=on
  Memory2 : Memory
  NOT : Logic  Operator=NOT  IconShape=distinctive  AllPortsSameDT=off  OutDataTypeStr=boolean
  Product : Product
  Product1 : Product
  Pulse Generator5 : DiscretePulseGenerator  PulseType=Time based  Period=Th_control_time2  PulseWidth=0.00001/Th_control_time2*100  PhaseDelay=Th_control_time2
  Scope1 : Scope  NumInputPorts=3
  Scope2 : Scope  NumInputPorts=3
  Scope3 : Scope  NumInputPorts=3
  Scope4 : Scope  NumInputPorts=4
  Sum : Sum  Inputs=++|
  Sum1 : Sum  Inputs=|++
  Switch3 : Switch  Criteria=u2 > Threshold  SaturateOnIntegerOverflow=off  InputSameDT=off
  Switch4 : Switch  Threshold=Th_plus_count2  SaturateOnIntegerOverflow=off  InputSameDT=off
  Switch5 : Switch  Threshold=Th_minus_count2  SaturateOnIntegerOverflow=off  InputSameDT=off
  spike_generator2 : Subsystem
  Threshold : Outport
  wires:
  MATLAB Function2/1(y) -> Scope3/1, Sum/2
  Sum/1 -> MATLAB Function/1(u)  "Threshold"
  From Workspace7/1 -> MATLAB Function/3(max)
  Delay1/1 -> Scope3/3, MATLAB Function2/3(before_threshold)
  neuron_num/1 -> MATLAB Function2/2(neuron_num)
  MATLAB Function/1(y) -> Delay1/1, Scope3/2, Threshold/1
  initial_threshold/1 -> MATLAB Function2/1(init_th)
  From Workspace6/1 -> MATLAB Function/2(min)
  Pulse Generator5/1 -> Switch3/2, Scope4/1, Product1/1, NOT/1
  Product1/1 -> Scope2/2, Scope4/2, spike_generator2/1(del_th)
  spike/1 -> Scope2/1, Sum1/1
  Delay/1 -> Sum1/2
  Product/1 -> Delay/1, Scope2/3
  Switch4/1 -> Add1/1, Scope1/1
  Switch5/1 -> Scope1/3, Add1/2
  Sum1/1 -> Product1/2, Product/2
  Constant2/1 -> Switch5/1, Switch4/3
  From Workspace4/1 -> Switch5/3
  Switch3/1 -> Scope4/4, Switch5/2, Switch4/2
  From Workspace3/1 -> Switch4/1
  NOT/1 -> Product/1
  spike_generator2/1(del_th_spike) -> Switch3/1, Scope4/3
  From Workspace5/1 -> Switch3/3
  Memory2/1 -> Scope1/2, Sum/1
  Add1/1 -> Memory2/1

== system pattern3x3_training_2023noclock/Neuron2/spike_generator1 ==
  1 : Inport
  AND : Logic  IconShape=distinctive  AllPortsSameDT=off  OutDataTypeStr=boolean
  Cast To Double : DataTypeConversion  OutDataTypeStr=double  SaturateOnIntegerOverflow=off  RndMeth=Floor
  Delay1 : Delay
  NOT : Logic  Operator=NOT  IconShape=distinctive  AllPortsSameDT=off  OutDataTypeStr=boolean
  Scope3 : Scope  NumInputPorts=5
  spike : Outport
  wires:
  NOT/1 -> Scope3/2, Delay1/1
  Delay1/1 -> Scope3/3, AND/2
  AND/1 -> Scope3/4, Cast To Double/1
  1/1 -> AND/1, Scope3/1, NOT/1
  Cast To Double/1 -> Scope3/5, spike/1

== system pattern3x3_training_2023noclock/Neuron3/Clock4 ==
  "Reset " : Inport
  Memory2 : Memory
  NOT1 : Logic  Operator=NOT  IconShape=distinctive  AllPortsSameDT=off  OutDataTypeStr=boolean
  Product1 : Product
  Pulse Generator1 : DiscretePulseGenerator  PulseType=Time based  Period=0.00001  PulseWidth=50
  Triggered Subsystem1 : Subsystem  TreatAsAtomicUnit=on
  T : Outport  VectorParamsAs1DForOutWhenUnconnected=off
  wires:
  Memory2/1 -> Triggered Subsystem1/1(In1)
  Product1/1 -> T/1, Memory2/1
  Pulse Generator1/1 -> Triggered Subsystem1/Trigger
  "Reset "/1 -> NOT1/1
  Triggered Subsystem1/1(Out1) -> Product1/1
  NOT1/1 -> Product1/2

== system pattern3x3_training_2023noclock/Neuron3/Clock5 ==
  "Reset " : Inport
  Memory2 : Memory
  NOT1 : Logic  Operator=NOT  IconShape=distinctive  AllPortsSameDT=off  OutDataTypeStr=boolean
  Product1 : Product
  Pulse Generator1 : DiscretePulseGenerator  PulseType=Time based  Period=0.00001  PulseWidth=50
  Triggered Subsystem1 : Subsystem  TreatAsAtomicUnit=on
  T : Outport  VectorParamsAs1DForOutWhenUnconnected=off
  wires:
  Memory2/1 -> Triggered Subsystem1/1(In1)
  Product1/1 -> T/1, Memory2/1
  Pulse Generator1/1 -> Triggered Subsystem1/Trigger
  "Reset "/1 -> NOT1/1
  Triggered Subsystem1/1(Out1) -> Product1/1
  NOT1/1 -> Product1/2

== system pattern3x3_training_2023noclock/Neuron3/Subsystem2 ==
  note: 기존 membrane potential + input potential
  Input potential : Inport
  before_Potential : Inport  Port=2
  Trigger : TriggerPort  VariantControl=(inherit)  PortDimensions=1
  Sum : Sum  Inputs=|++
  membrane_state : Outport
  wires:
  Input potential/1 -> Sum/1
  Sum/1 -> membrane_state/1
  before_Potential/1 -> Sum/2

== system pattern3x3_training_2023noclock/Neuron3/Subsystem3 ==
  spike : Inport  OutDataTypeStr=double
  initial_threshold : Inport  Port=2
  neuron_num : Inport  Port=3
  Add1 : Sum
  Constant2 : Constant  Value=0
  Delay : Delay  DelayLength=1  SampleTime=0.00001
  Delay1 : Delay  DelayLength=1  SampleTime=0.00001
  From Workspace3 : FromWorkspace  VariableName=Th_plus
  From Workspace4 : FromWorkspace  VariableName=Th_minus
  From Workspace5 : FromWorkspace  VariableName=Th_mean_count
  From Workspace6 : FromWorkspace  VariableName=min_th
  From Workspace7 : FromWorkspace  VariableName=max_th
  MATLAB Function : MATLAB Function  TreatAsAtomicUnit=on
  MATLAB Function2 : MATLAB Function  TreatAsAtomicUnit=on
  Memory2 : Memory
  NOT : Logic  Operator=NOT  IconShape=distinctive  AllPortsSameDT=off  OutDataTypeStr=boolean
  Product : Product
  Product1 : Product
  Pulse Generator5 : DiscretePulseGenerator  PulseType=Time based  Period=Th_control_time2  PulseWidth=0.00001/Th_control_time2*100  PhaseDelay=Th_control_time2
  Scope1 : Scope  NumInputPorts=3
  Scope2 : Scope  NumInputPorts=3
  Scope3 : Scope  NumInputPorts=3
  Scope4 : Scope  NumInputPorts=4
  Sum : Sum  Inputs=++|
  Sum1 : Sum  Inputs=|++
  Switch3 : Switch  Criteria=u2 > Threshold  SaturateOnIntegerOverflow=off  InputSameDT=off
  Switch4 : Switch  Threshold=Th_plus_count2  SaturateOnIntegerOverflow=off  InputSameDT=off
  Switch5 : Switch  Threshold=Th_minus_count2  SaturateOnIntegerOverflow=off  InputSameDT=off
  spike_generator2 : Subsystem
  Threshold : Outport
  wires:
  MATLAB Function2/1(y) -> Scope3/1, Sum/2
  Sum/1 -> MATLAB Function/1(u)  "Threshold"
  From Workspace7/1 -> MATLAB Function/3(max)
  Delay1/1 -> Scope3/3, MATLAB Function2/3(before_threshold)
  neuron_num/1 -> MATLAB Function2/2(neuron_num)
  MATLAB Function/1(y) -> Delay1/1, Scope3/2, Threshold/1
  initial_threshold/1 -> MATLAB Function2/1(init_th)
  From Workspace6/1 -> MATLAB Function/2(min)
  Pulse Generator5/1 -> Switch3/2, Scope4/1, Product1/1, NOT/1
  Product1/1 -> Scope2/2, Scope4/2, spike_generator2/1(del_th)
  spike/1 -> Scope2/1, Sum1/1
  Delay/1 -> Sum1/2
  Product/1 -> Delay/1, Scope2/3
  Switch4/1 -> Add1/1, Scope1/1
  Switch5/1 -> Scope1/3, Add1/2
  Sum1/1 -> Product1/2, Product/2
  Constant2/1 -> Switch5/1, Switch4/3
  From Workspace4/1 -> Switch5/3
  Switch3/1 -> Scope4/4, Switch5/2, Switch4/2
  From Workspace3/1 -> Switch4/1
  NOT/1 -> Product/1
  spike_generator2/1(del_th_spike) -> Switch3/1, Scope4/3
  From Workspace5/1 -> Switch3/3
  Memory2/1 -> Scope1/2, Sum/1
  Add1/1 -> Memory2/1

== system pattern3x3_training_2023noclock/Neuron3/spike_generator1 ==
  1 : Inport
  AND : Logic  IconShape=distinctive  AllPortsSameDT=off  OutDataTypeStr=boolean
  Cast To Double : DataTypeConversion  OutDataTypeStr=double  SaturateOnIntegerOverflow=off  RndMeth=Floor
  Delay1 : Delay
  NOT : Logic  Operator=NOT  IconShape=distinctive  AllPortsSameDT=off  OutDataTypeStr=boolean
  Scope3 : Scope  NumInputPorts=5
  spike : Outport
  wires:
  NOT/1 -> Scope3/2, Delay1/1
  Delay1/1 -> Scope3/3, AND/2
  AND/1 -> Scope3/4, Cast To Double/1
  1/1 -> AND/1, Scope3/1, NOT/1
  Cast To Double/1 -> Scope3/5, spike/1

== system pattern3x3_training_2023noclock/Neuron4/Clock4 ==
  "Reset " : Inport
  Memory2 : Memory
  NOT1 : Logic  Operator=NOT  IconShape=distinctive  AllPortsSameDT=off  OutDataTypeStr=boolean
  Product1 : Product
  Pulse Generator1 : DiscretePulseGenerator  PulseType=Time based  Period=0.00001  PulseWidth=50
  Triggered Subsystem1 : Subsystem  TreatAsAtomicUnit=on
  T : Outport  VectorParamsAs1DForOutWhenUnconnected=off
  wires:
  Memory2/1 -> Triggered Subsystem1/1(In1)
  Product1/1 -> T/1, Memory2/1
  Pulse Generator1/1 -> Triggered Subsystem1/Trigger
  "Reset "/1 -> NOT1/1
  Triggered Subsystem1/1(Out1) -> Product1/1
  NOT1/1 -> Product1/2

== system pattern3x3_training_2023noclock/Neuron4/Clock5 ==
  "Reset " : Inport
  Memory2 : Memory
  NOT1 : Logic  Operator=NOT  IconShape=distinctive  AllPortsSameDT=off  OutDataTypeStr=boolean
  Product1 : Product
  Pulse Generator1 : DiscretePulseGenerator  PulseType=Time based  Period=0.00001  PulseWidth=50
  Triggered Subsystem1 : Subsystem  TreatAsAtomicUnit=on
  T : Outport  VectorParamsAs1DForOutWhenUnconnected=off
  wires:
  Memory2/1 -> Triggered Subsystem1/1(In1)
  Product1/1 -> T/1, Memory2/1
  Pulse Generator1/1 -> Triggered Subsystem1/Trigger
  "Reset "/1 -> NOT1/1
  Triggered Subsystem1/1(Out1) -> Product1/1
  NOT1/1 -> Product1/2

== system pattern3x3_training_2023noclock/Neuron4/Subsystem2 ==
  note: 기존 membrane potential + input potential
  Input potential : Inport
  before_Potential : Inport  Port=2
  Trigger : TriggerPort  VariantControl=(inherit)  PortDimensions=1
  Sum : Sum  Inputs=|++
  membrane_state : Outport
  wires:
  Input potential/1 -> Sum/1
  Sum/1 -> membrane_state/1
  before_Potential/1 -> Sum/2

== system pattern3x3_training_2023noclock/Neuron4/Subsystem3 ==
  spike : Inport  OutDataTypeStr=double
  initial_threshold : Inport  Port=2
  neuron_num : Inport  Port=3
  Add1 : Sum
  Constant2 : Constant  Value=0
  Delay : Delay  DelayLength=1  SampleTime=0.00001
  Delay1 : Delay  DelayLength=1  SampleTime=0.00001
  From Workspace3 : FromWorkspace  VariableName=Th_plus
  From Workspace4 : FromWorkspace  VariableName=Th_minus
  From Workspace5 : FromWorkspace  VariableName=Th_mean_count
  From Workspace6 : FromWorkspace  VariableName=min_th
  From Workspace7 : FromWorkspace  VariableName=max_th
  MATLAB Function : MATLAB Function  TreatAsAtomicUnit=on
  MATLAB Function2 : MATLAB Function  TreatAsAtomicUnit=on
  Memory2 : Memory
  NOT : Logic  Operator=NOT  IconShape=distinctive  AllPortsSameDT=off  OutDataTypeStr=boolean
  Product : Product
  Product1 : Product
  Pulse Generator5 : DiscretePulseGenerator  PulseType=Time based  Period=Th_control_time2  PulseWidth=0.00001/Th_control_time2*100  PhaseDelay=Th_control_time2
  Scope1 : Scope  NumInputPorts=3
  Scope2 : Scope  NumInputPorts=3
  Scope3 : Scope  NumInputPorts=3
  Scope4 : Scope  NumInputPorts=4
  Sum : Sum  Inputs=++|
  Sum1 : Sum  Inputs=|++
  Switch3 : Switch  Criteria=u2 > Threshold  SaturateOnIntegerOverflow=off  InputSameDT=off
  Switch4 : Switch  Threshold=Th_plus_count2  SaturateOnIntegerOverflow=off  InputSameDT=off
  Switch5 : Switch  Threshold=Th_minus_count2  SaturateOnIntegerOverflow=off  InputSameDT=off
  spike_generator2 : Subsystem
  Threshold : Outport
  wires:
  MATLAB Function2/1(y) -> Scope3/1, Sum/2
  Sum/1 -> MATLAB Function/1(u)  "Threshold"
  From Workspace7/1 -> MATLAB Function/3(max)
  Delay1/1 -> Scope3/3, MATLAB Function2/3(before_threshold)
  neuron_num/1 -> MATLAB Function2/2(neuron_num)
  MATLAB Function/1(y) -> Delay1/1, Scope3/2, Threshold/1
  initial_threshold/1 -> MATLAB Function2/1(init_th)
  From Workspace6/1 -> MATLAB Function/2(min)
  Pulse Generator5/1 -> Switch3/2, Scope4/1, Product1/1, NOT/1
  Product1/1 -> Scope2/2, Scope4/2, spike_generator2/1(del_th)
  spike/1 -> Scope2/1, Sum1/1
  Delay/1 -> Sum1/2
  Product/1 -> Delay/1, Scope2/3
  Switch4/1 -> Add1/1, Scope1/1
  Switch5/1 -> Scope1/3, Add1/2
  Sum1/1 -> Product1/2, Product/2
  Constant2/1 -> Switch5/1, Switch4/3
  From Workspace4/1 -> Switch5/3
  Switch3/1 -> Scope4/4, Switch5/2, Switch4/2
  From Workspace3/1 -> Switch4/1
  NOT/1 -> Product/1
  spike_generator2/1(del_th_spike) -> Switch3/1, Scope4/3
  From Workspace5/1 -> Switch3/3
  Memory2/1 -> Scope1/2, Sum/1
  Add1/1 -> Memory2/1

== system pattern3x3_training_2023noclock/Neuron4/spike_generator1 ==
  1 : Inport
  AND : Logic  IconShape=distinctive  AllPortsSameDT=off  OutDataTypeStr=boolean
  Cast To Double : DataTypeConversion  OutDataTypeStr=double  SaturateOnIntegerOverflow=off  RndMeth=Floor
  Delay1 : Delay
  NOT : Logic  Operator=NOT  IconShape=distinctive  AllPortsSameDT=off  OutDataTypeStr=boolean
  Scope3 : Scope  NumInputPorts=5
  spike : Outport
  wires:
  NOT/1 -> Scope3/2, Delay1/1
  Delay1/1 -> Scope3/3, AND/2
  AND/1 -> Scope3/4, Cast To Double/1
  1/1 -> AND/1, Scope3/1, NOT/1
  Cast To Double/1 -> Scope3/5, spike/1

== system pattern3x3_training_2023noclock/Neuron5/Clock4 ==
  "Reset " : Inport
  Memory2 : Memory
  NOT1 : Logic  Operator=NOT  IconShape=distinctive  AllPortsSameDT=off  OutDataTypeStr=boolean
  Product1 : Product
  Pulse Generator1 : DiscretePulseGenerator  PulseType=Time based  Period=0.00001  PulseWidth=50
  Triggered Subsystem1 : Subsystem  TreatAsAtomicUnit=on
  T : Outport  VectorParamsAs1DForOutWhenUnconnected=off
  wires:
  Memory2/1 -> Triggered Subsystem1/1(In1)
  Product1/1 -> T/1, Memory2/1
  Pulse Generator1/1 -> Triggered Subsystem1/Trigger
  "Reset "/1 -> NOT1/1
  Triggered Subsystem1/1(Out1) -> Product1/1
  NOT1/1 -> Product1/2

== system pattern3x3_training_2023noclock/Neuron5/Clock5 ==
  "Reset " : Inport
  Memory2 : Memory
  NOT1 : Logic  Operator=NOT  IconShape=distinctive  AllPortsSameDT=off  OutDataTypeStr=boolean
  Product1 : Product
  Pulse Generator1 : DiscretePulseGenerator  PulseType=Time based  Period=0.00001  PulseWidth=50
  Triggered Subsystem1 : Subsystem  TreatAsAtomicUnit=on
  T : Outport  VectorParamsAs1DForOutWhenUnconnected=off
  wires:
  Memory2/1 -> Triggered Subsystem1/1(In1)
  Product1/1 -> T/1, Memory2/1
  Pulse Generator1/1 -> Triggered Subsystem1/Trigger
  "Reset "/1 -> NOT1/1
  Triggered Subsystem1/1(Out1) -> Product1/1
  NOT1/1 -> Product1/2

== system pattern3x3_training_2023noclock/Neuron5/Subsystem2 ==
  note: 기존 membrane potential + input potential
  Input potential : Inport
  before_Potential : Inport  Port=2
  Trigger : TriggerPort  VariantControl=(inherit)  PortDimensions=1
  Sum : Sum  Inputs=|++
  membrane_state : Outport
  wires:
  Input potential/1 -> Sum/1
  Sum/1 -> membrane_state/1
  before_Potential/1 -> Sum/2
